simulink model "TestMassAccelerometer_NonlinearModel_LQR_KF_Simulink2017"  (R2018b)
settings: Solver=ode4  StartTime=0.0  StopTime=SIM_TIME  FixedStep=STEP_SIZE  RelTol=1e-3
undefined symbols (not defined in the file): A0, A1, c1, c2, C_kf, f1, f2, f3, f4, f5, f6, F_kf, g, G_kf, Iss, K_lqr_fs, K_lqr_int, L_kf, m, STEP_TIME, Ts, V2, x0, x0_hat, x0_int, X_ref, Xss
settings Model: Creator=Roberto  LastModifiedBy=Roberto
settings SFSimCC: SimUseLocalCustomCode=off
settings RTWCC: RTWUseLocalCustomCode=off
settings CodeAppCC: StateflowObjectComments=on

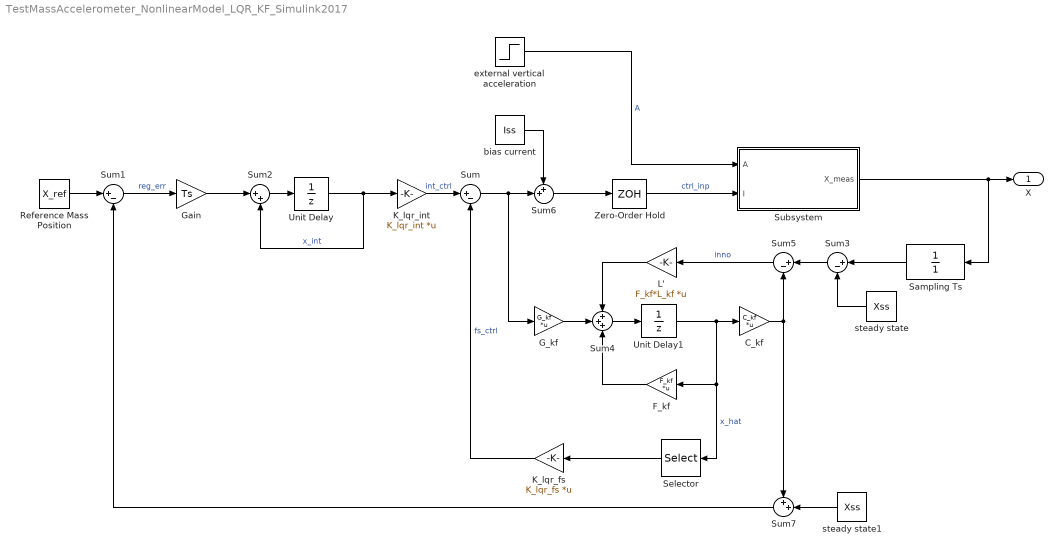
== system TestMassAccelerometer_NonlinearModel_LQR_KF_Simulink2017 ==
  C_kf : Gain  Gain=C_kf  Multiplication=Matrix(K*u) (u vector)
  F_kf : Gain  Gain=F_kf  Multiplication=Matrix(K*u) (u vector)
  G_kf : Gain  Gain=G_kf  Multiplication=Matrix(K*u) (u vector)
  Gain : Gain  Gain=Ts
  K_lqr_fs : Gain  Gain=K_lqr_fs  Multiplication=Matrix(K*u) (u vector)
  K_lqr_int : Gain  Gain=K_lqr_int  Multiplication=Matrix(K*u) (u vector)
  L' : Gain  Gain=F_kf*L_kf  Multiplication=Matrix(K*u) (u vector)
  Reference Mass Position : Constant  Value=X_ref
  Sampling Ts : DiscreteTransferFcn  Denominator=[1]  SampleTime=Ts
  Selector : Selector  InputPortWidth=3  IndexOptions=Index vector (dialog)  Indices=[1 2]  OutputSizes=1
  Subsystem : Subsystem
  Sum{,1,3,5} (4 alike) : Sum  Inputs=|+-
  Sum2 : Sum  Inputs=|++
  Sum4 : Sum  Inputs=+++
  Sum6 : Sum  Inputs=++|
  Sum7 : Sum  Inputs=++|
  Unit Delay : UnitDelay  InitialCondition=x0_int  SampleTime=Ts
  Unit Delay1 : UnitDelay  InitialCondition=x0_hat  SampleTime=Ts
  Zero-Order Hold : ZeroOrderHold  SampleTime=Ts
  bias current : Constant  Value=Iss
  external vertical acceleration : Step  Time=STEP_TIME  Before=A0  After=A1  SampleTime=0
  steady state : Constant  Value=Xss
  steady state1 : Constant  Value=Xss
  X : Outport
  wires:
  Zero-Order Hold/1 -> Subsystem/2(I)  "ctrl_inp"
  K_lqr_fs/1 -> Sum/2  "fs_ctrl"
  Reference Mass Position/1 -> Sum1/1
  Subsystem/1(X_meas) -> Sampling Ts/1, X/1
  Sum2/1 -> Unit Delay/1
  Sum1/1 -> Gain/1  "reg_err"
  Unit Delay/1 -> Sum2/2, K_lqr_int/1  "x_int"
  steady state/1 -> Sum3/2
  external vertical acceleration/1 -> Subsystem/1(A)  "A"
  Sum4/1 -> Unit Delay1/1
  F_kf/1 -> Sum4/3
  Unit Delay1/1 -> Selector/1, F_kf/1, C_kf/1  "x_hat"
  G_kf/1 -> Sum4/2
  L'/1 -> Sum4/1
  Sum5/1 -> L'/1  "inno"
  Selector/1 -> K_lqr_fs/1
  C_kf/1 -> Sum5/2, Sum7/1
  K_lqr_int/1 -> Sum/1  "int_ctrl"
  Sum/1 -> G_kf/1, Sum6/2
  Sum6/1 -> Zero-Order Hold/1
  bias current/1 -> Sum6/1
  steady state1/1 -> Sum7/2
  Sum7/1 -> Sum1/2
  Gain/1 -> Sum2/1
  Sampling Ts/1 -> Sum3/1
  Sum3/1 -> Sum5/1

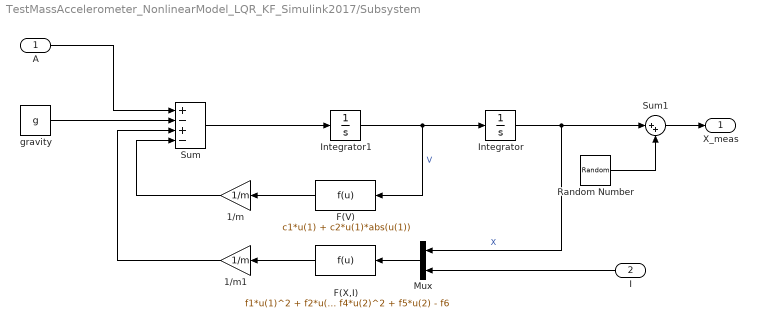
== system TestMassAccelerometer_NonlinearModel_LQR_KF_Simulink2017/Subsystem ==
  A : Inport
  I : Inport  Port=2
  1/m : Gain  Gain=1/m
  1/m1 : Gain  Gain=1/m
  F(V) : Fcn  Expr=c1*u(1) + c2*u(1)*abs(u(1))
  F(X,I) : Fcn  Expr=f1*u(1)^2 + f2*u(1)*u(2) - f3*u(1) + f4*u(2)^2 + f5*u(2) - f6
  Integrator : Integrator  Priority=1  InitialCondition=x0(1)
  Integrator1 : Integrator  Priority=2  InitialCondition=x0(2)
  Mux : Mux  Inputs=2
  Random Number : RandomNumber  Variance=V2  Seed=318569  SampleTime=Ts
  Sum : Sum  Inputs=+-+-
  Sum1 : Sum  Inputs=|++
  gravity : Constant  Value=g
  X_meas : Outport
  wires:
  I/1 -> Mux/2
  Integrator1/1 -> Integrator/1, F(V)/1  "V"
  Sum/1 -> Integrator1/1
  gravity/1 -> Sum/2
  A/1 -> Sum/1
  Mux/1 -> F(X,I)/1
  Integrator/1 -> Sum1/1, Mux/1  "X"
  F(X,I)/1 -> 1/m1/1
  F(V)/1 -> 1/m/1
  1/m/1 -> Sum/4
  1/m1/1 -> Sum/3
  Sum1/1 -> X_meas/1
  Random Number/1 -> Sum1/2
